simulink model "sampleModel7288_pp_1_1"  (R2018a)
settings: Solver=VariableStepAuto  StartTime=0.0  StopTime=10.0  RelTol=1e-3
undefined symbols (not defined in the file): DiscIntNeverNeededParam, sigbuilder_block
libraries: simulink x497
(part 2 of 10)

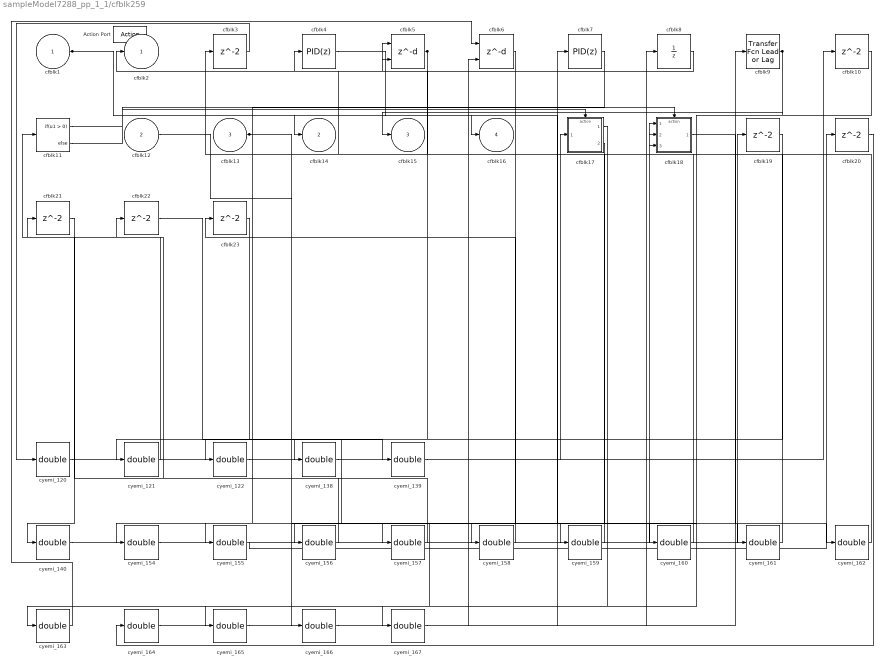
== system sampleModel7288_pp_1_1/cfblk259 ==
  cfblk1 : Inport
  cfblk12 : Inport  Port=2
  cfblk13 : Inport  Port=3
  Action Port : ActionPort  ActionType=else
  cfblk{3,10,19..23} (7 alike) : Delay
  cfblk11 : If  SampleTime=1
  cfblk17 : Subsystem  TreatAsAtomicUnit=on
  cfblk18 : Subsystem  TreatAsAtomicUnit=on
  cfblk4 : simulink/Continuous/PID Controller  Controller=PID  TimeDomain=Discrete-time  SampleTime=-1  IntegratorMethod=Forward Euler  FilterMethod=Forward Euler  Form=Parallel  UseFilter=on  ControllerParametersSource=internal  P=1  I=1  D=0  N=100  InitialConditionSource=internal  InitialConditionForIntegrator=0  InitialConditionForFilter=0  ExternalReset=none  LimitOutput=off  UpperSaturationLimit=inf  LowerSaturationLimit=-inf  LinearizeAsGain=off  AntiWindupMode=none  Kb=1  TrackingMode=off  Kt=1  PParamMin=[]  PParamMax=[]  IParamMin=[]  IParamMax=[]  DParamMin=[]  DParamMax=[]  NParamMin=[]  NParamMax=[]  KbParamMin=[]  KbParamMax=[]  KtParamMin=[]  KtParamMax=[]  POutMin=[]  POutMax=[]  IOutMin=[]  IOutMax=[]  DOutMin=[]  DOutMax=[]  NOutMin=[]  NOutMax=[]  KbOutMin=[]  KbOutMax=[]  KtOutMin=[]  KtOutMax=[]  IntegratorOutMin=[]  IntegratorOutMax=[]  FilterOutMin=[]  FilterOutMax=[]  SumOutMin=[]  SumOutMax=[]  SumI1OutMin=[]  SumI1OutMax=[]  SumI2OutMin=[]  SumI2OutMax=[]  SumI3OutMin=[]  SumI3OutMax=[]  SumDOutMin=[]  SumDOutMax=[]  SaturationOutMin=[]  SaturationOutMax=[]  IntegratorContinuousStateAttributes=''  IntegratorStateMustResolveToSignalObject=off  IntegratorRTWStateStorageClass=Auto  FilterContinuousStateAttributes=''  FilterStateMustResolveToSignalObject=off  FilterRTWStateStorageClass=Auto  DifferentiatorICPrevScaledInput=0  DifferentiatorOutMin=[]  DifferentiatorOutMax=[]  FilterDiffOutCoefMin=[]  FilterDiffOutCoefMax=[]  SumDenOutMin=[]  SumDenOutMax=[]  SumNumOutMin=[]  SumNumOutMax=[]  ReciprocalOutMin=[]  ReciprocalOutMax=[]  DivideOutMin=[]  DivideOutMax=[]  TunerSelectOption=Transfer Function Based (PID Tuner App)
  cfblk5 : Delay  DelayLengthSource=Input port
      settings: InputPortMap=u0,p1
  cfblk6 : Delay  DelayLengthSource=Input port
      settings: InputPortMap=u0,p1
  cfblk7 : simulink/Continuous/PID Controller  Controller=PID  TimeDomain=Discrete-time  SampleTime=-1  IntegratorMethod=Forward Euler  FilterMethod=Forward Euler  Form=Parallel  UseFilter=on  ControllerParametersSource=internal  P=1  I=1  D=0  N=100  InitialConditionSource=internal  InitialConditionForIntegrator=0  InitialConditionForFilter=0  ExternalReset=none  LimitOutput=off  UpperSaturationLimit=inf  LowerSaturationLimit=-inf  LinearizeAsGain=off  AntiWindupMode=none  Kb=1  TrackingMode=off  Kt=1  PParamMin=[]  PParamMax=[]  IParamMin=[]  IParamMax=[]  DParamMin=[]  DParamMax=[]  NParamMin=[]  NParamMax=[]  KbParamMin=[]  KbParamMax=[]  KtParamMin=[]  KtParamMax=[]  POutMin=[]  POutMax=[]  IOutMin=[]  IOutMax=[]  DOutMin=[]  DOutMax=[]  NOutMin=[]  NOutMax=[]  KbOutMin=[]  KbOutMax=[]  KtOutMin=[]  KtOutMax=[]  IntegratorOutMin=[]  IntegratorOutMax=[]  FilterOutMin=[]  FilterOutMax=[]  SumOutMin=[]  SumOutMax=[]  SumI1OutMin=[]  SumI1OutMax=[]  SumI2OutMin=[]  SumI2OutMax=[]  SumI3OutMin=[]  SumI3OutMax=[]  SumDOutMin=[]  SumDOutMax=[]  SaturationOutMin=[]  SaturationOutMax=[]  IntegratorContinuousStateAttributes=''  IntegratorStateMustResolveToSignalObject=off  IntegratorRTWStateStorageClass=Auto  FilterContinuousStateAttributes=''  FilterStateMustResolveToSignalObject=off  FilterRTWStateStorageClass=Auto  DifferentiatorICPrevScaledInput=0  DifferentiatorOutMin=[]  DifferentiatorOutMax=[]  FilterDiffOutCoefMin=[]  FilterDiffOutCoefMax=[]  SumDenOutMin=[]  SumDenOutMax=[]  SumNumOutMin=[]  SumNumOutMax=[]  ReciprocalOutMin=[]  ReciprocalOutMax=[]  DivideOutMin=[]  DivideOutMax=[]  TunerSelectOption=Transfer Function Based (PID Tuner App)
  cfblk8 : UnitDelay  SampleTime=-1
  cfblk9 : simulink/Discrete/Transfer Fcn Lead or Lag  PoleZ=0.95  ZeroZ=0.75  ICPrevOutput=0.0  ICPrevInput=0.0  DoSatur=off
      settings: SourceProductName=Simulink  SourceProductBaseCode=SL
  cyemi_{120..122,138..140,154..167} (20 alike) : DataTypeConversion  OutDataTypeStr=double
  cfblk2 : Outport
  cfblk14 : Outport  Port=2
  cfblk15 : Outport  Port=3
  cfblk16 : Outport  Port=4
  wires:
  cfblk13/1 -> cyemi_159/1, cyemi_160/1
  cfblk8/1 -> cfblk2/1
  cfblk9/1 -> cfblk15/1, cyemi_154/1, cyemi_157/1
  cfblk5/1 -> cyemi_155/1, cyemi_156/1
  cfblk1/1 -> cfblk14/1, cfblk16/1
  cfblk11/1 -> cfblk17/Action
  cfblk11/2 -> cfblk18/Action
  cyemi_120/1 -> cfblk10/1
  cfblk3/1 -> cyemi_120/1
  cyemi_121/1 -> cfblk11/1
  cfblk23/1 -> cyemi_121/1
  cyemi_122/1 -> cfblk17/1(cfblk1)
  cfblk7/1 -> cyemi_122/1
  cyemi_138/1 -> cfblk18/1(cfblk1)
  cfblk19/1 -> cyemi_138/1
  cyemi_139/1 -> cfblk18/2(cfblk12)
  cfblk22/1 -> cyemi_139/1
  cyemi_140/1 -> cfblk18/3(cfblk13)
  cfblk21/1 -> cyemi_140/1
  cyemi_154/1 -> cfblk19/1
  cyemi_155/1 -> cfblk20/1
  cyemi_156/1 -> cfblk21/1
  cyemi_157/1 -> cfblk22/1
  cyemi_158/1 -> cfblk23/1
  cfblk17/2(cfblk11) -> cyemi_158/1
  cyemi_159/1 -> cfblk3/1
  cyemi_160/1 -> cfblk4/1
  cyemi_161/1 -> cfblk5/1
  cfblk4/1 -> cyemi_161/1
  cyemi_162/1 -> cfblk5/2
  cfblk18/1(cfblk2) -> cyemi_162/1
  cyemi_163/1 -> cfblk6/1
  cfblk17/1(cfblk2) -> cyemi_163/1
  cyemi_164/1 -> cfblk6/2
  cfblk20/1 -> cyemi_164/1
  cyemi_165/1 -> cfblk7/1
  cfblk10/1 -> cyemi_165/1
  cyemi_166/1 -> cfblk8/1
  cfblk12/1 -> cyemi_166/1
  cyemi_167/1 -> cfblk9/1
  cfblk6/1 -> cyemi_167/1

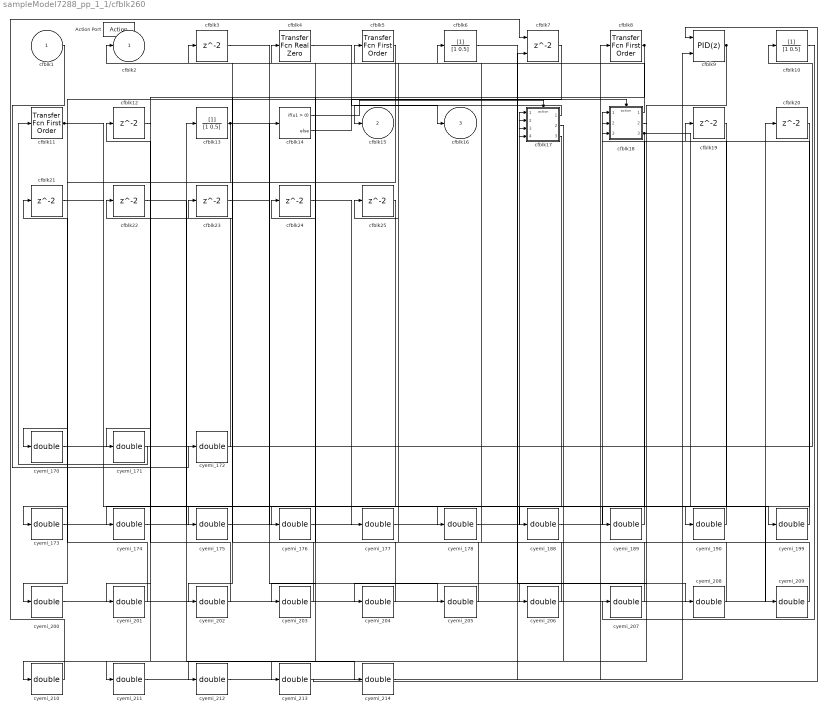
== system sampleModel7288_pp_1_1/cfblk260 ==
  cfblk1 : Inport
  Action Port : ActionPort  ActionType=then
  cfblk10 : DiscreteFilter
  cfblk11 : simulink/Discrete/Transfer Fcn First Order  PoleZ=0.95  ICPrevOutput=0.0  DoSatur=off
      settings: SourceProductName=Simulink
  cfblk{3,12,19..25} (9 alike) : Delay
  cfblk13 : DiscreteFilter
  cfblk14 : If  SampleTime=1
  cfblk17 : Subsystem  TreatAsAtomicUnit=on
  cfblk18 : Subsystem  TreatAsAtomicUnit=on
  cfblk4 : simulink/Discrete/Transfer Fcn Real Zero  ZeroZ=0.75  ICPrevInput=0.0  DoSatur=off
      settings: SourceProductName=Simulink  SourceProductBaseCode=SL
  cfblk5 : simulink/Discrete/Transfer Fcn First Order  PoleZ=0.95  ICPrevOutput=0.0  DoSatur=off
      settings: SourceProductName=Simulink
  cfblk6 : DiscreteFilter
  cfblk7 : Delay  ShowEnablePort=on
      settings: InputPortMap=u0,e6
  cfblk8 : simulink/Discrete/Transfer Fcn First Order  PoleZ=0.95  ICPrevOutput=0.0  DoSatur=off
      settings: SourceProductName=Simulink
  cfblk9 : simulink/Continuous/PID Controller (2DOF)  Controller=PID  TimeDomain=Discrete-time  SampleTime=-1  IntegratorMethod=Forward Euler  FilterMethod=Forward Euler  Form=Parallel  UseFilter=on  ControllerParametersSource=internal  P=1  I=1  D=0  N=100  b=1  c=1  InitialConditionSource=internal  InitialConditionForIntegrator=0  InitialConditionForFilter=0  ExternalReset=none  LimitOutput=off  UpperSaturationLimit=inf  LowerSaturationLimit=-inf  LinearizeAsGain=off  AntiWindupMode=none  Kb=1  TrackingMode=off  Kt=1  PParamMin=[]  PParamMax=[]  IParamMin=[]  IParamMax=[]  DParamMin=[]  DParamMax=[]  NParamMin=[]  NParamMax=[]  bParamMin=[]  bParamMax=[]  cParamMin=[]  cParamMax=[]  KbParamMin=[]  KbParamMax=[]  KtParamMin=[]  KtParamMax=[]  POutMin=[]  POutMax=[]  IOutMin=[]  IOutMax=[]  DOutMin=[]  DOutMax=[]  NOutMin=[]  NOutMax=[]  bOutMin=[]  bOutMax=[]  cOutMin=[]  cOutMax=[]  KbOutMin=[]  KbOutMax=[]  KtOutMin=[]  KtOutMax=[]  IntegratorOutMin=[]  IntegratorOutMax=[]  FilterOutMin=[]  FilterOutMax=[]  SumOutMin=[]  SumOutMax=[]  Sum1OutMin=[]  Sum1OutMax=[]  Sum2OutMin=[]  Sum2OutMax=[]  Sum3OutMin=[]  Sum3OutMax=[]  SumI1OutMin=[]  SumI1OutMax=[]  SumI2OutMin=[]  SumI2OutMax=[]  SumI3OutMin=[]  SumI3OutMax=[]  SumDOutMin=[]  SumDOutMax=[]  SaturationOutMin=[]  SaturationOutMax=[]  IntegratorContinuousStateAttributes=''  IntegratorStateMustResolveToSignalObject=off  IntegratorRTWStateStorageClass=Auto  FilterContinuousStateAttributes=''  FilterStateMustResolveToSignalObject=off  FilterRTWStateStorageClass=Auto  DifferentiatorICPrevScaledInput=0  DifferentiatorOutMin=[]  DifferentiatorOutMax=[]  FilterDiffOutCoefMin=[]  FilterDiffOutCoefMax=[]  SumDenOutMin=[]  SumDenOutMax=[]  SumNumOutMin=[]  SumNumOutMax=[]  ReciprocalOutMin=[]  ReciprocalOutMax=[]  DivideOutMin=[]  DivideOutMax=[]  TunerSelectOption=Transfer Function Based (PID Tuner App)
  cyemi_{170..178,188..190,199..214} (28 alike) : DataTypeConversion  OutDataTypeStr=double
  cfblk2 : Outport
  cfblk15 : Outport  Port=2
  cfblk16 : Outport  Port=3
  wires:
  cfblk9/1 -> cyemi_204/1, cyemi_212/1
  cfblk11/1 -> cyemi_170/1, cyemi_189/1
  cfblk17/1(cfblk2) -> cfblk15/1
  cfblk8/1 -> cyemi_201/1, cyemi_202/1, cyemi_203/1
  cfblk13/1 -> cyemi_199/1, cyemi_200/1
  cfblk18/1(cfblk2) -> cfblk2/1
  cfblk4/1 -> cfblk16/1
  cfblk18/3(cfblk14) -> cyemi_206/1, cyemi_209/1
  cfblk14/1 -> cfblk17/Action
  cfblk14/2 -> cfblk18/Action
  cyemi_170/1 -> cfblk10/1
  cyemi_171/1 -> cfblk11/1
  cfblk12/1 -> cyemi_171/1
  cyemi_172/1 -> cfblk12/1
  cfblk1/1 -> cyemi_172/1
  cyemi_173/1 -> cfblk13/1
  cfblk7/1 -> cyemi_173/1
  cyemi_174/1 -> cfblk14/1
  cfblk25/1 -> cyemi_174/1
  cyemi_175/1 -> cfblk17/1(cfblk1)
  cfblk19/1 -> cyemi_175/1
  cyemi_176/1 -> cfblk17/2(cfblk10)
  cfblk18/2(cfblk13) -> cyemi_176/1
  cyemi_177/1 -> cfblk17/3(cfblk11)
  cfblk24/1 -> cyemi_177/1
  cyemi_178/1 -> cfblk17/4(cfblk12)
  cfblk23/1 -> cyemi_178/1
  cyemi_188/1 -> cfblk18/1(cfblk1)
  cfblk21/1 -> cyemi_188/1
  cyemi_189/1 -> cfblk18/2(cfblk11)
  cyemi_190/1 -> cfblk18/3(cfblk12)
  cfblk20/1 -> cyemi_190/1
  cyemi_199/1 -> cfblk19/1
  cyemi_200/1 -> cfblk20/1
  cyemi_201/1 -> cfblk21/1
  cyemi_202/1 -> cfblk22/1
  cyemi_203/1 -> cfblk23/1
  cyemi_204/1 -> cfblk24/1
  cyemi_205/1 -> cfblk25/1
  cfblk3/1 -> cyemi_205/1
  cyemi_206/1 -> cfblk3/1
  cyemi_207/1 -> cfblk4/1
  cfblk10/1 -> cyemi_207/1
  cyemi_208/1 -> cfblk5/1
  cfblk6/1 -> cyemi_208/1
  cyemi_209/1 -> cfblk6/1
  cyemi_210/1 -> cfblk7/1
  cfblk17/2(cfblk13) -> cyemi_210/1
  cyemi_211/1 -> cfblk7/2
  cfblk5/1 -> cyemi_211/1
  cyemi_212/1 -> cfblk8/1
  cyemi_213/1 -> cfblk9/1
  cfblk17/3(cfblk14) -> cyemi_213/1
  cyemi_214/1 -> cfblk9/2
  cfblk22/1 -> cyemi_214/1

== system sampleModel7288_pp_1_1/cfblk261 ==
  cfblk1 : Inport
  cfblk12 : Inport  Port=2
  Action Port : ActionPort  ActionType=else
  cfblk10 : simulink/Continuous/PID Controller  Controller=PID  TimeDomain=Discrete-time  SampleTime=-1  IntegratorMethod=Forward Euler  FilterMethod=Forward Euler  Form=Parallel  UseFilter=on  ControllerParametersSource=internal  P=1  I=1  D=0  N=100  InitialConditionSource=internal  InitialConditionForIntegrator=0  InitialConditionForFilter=0  ExternalReset=none  LimitOutput=off  UpperSaturationLimit=inf  LowerSaturationLimit=-inf  LinearizeAsGain=off  AntiWindupMode=none  Kb=1  TrackingMode=off  Kt=1  PParamMin=[]  PParamMax=[]  IParamMin=[]  IParamMax=[]  DParamMin=[]  DParamMax=[]  NParamMin=[]  NParamMax=[]  KbParamMin=[]  KbParamMax=[]  KtParamMin=[]  KtParamMax=[]  POutMin=[]  POutMax=[]  IOutMin=[]  IOutMax=[]  DOutMin=[]  DOutMax=[]  NOutMin=[]  NOutMax=[]  KbOutMin=[]  KbOutMax=[]  KtOutMin=[]  KtOutMax=[]  IntegratorOutMin=[]  IntegratorOutMax=[]  FilterOutMin=[]  FilterOutMax=[]  SumOutMin=[]  SumOutMax=[]  SumI1OutMin=[]  SumI1OutMax=[]  SumI2OutMin=[]  SumI2OutMax=[]  SumI3OutMin=[]  SumI3OutMax=[]  SumDOutMin=[]  SumDOutMax=[]  SaturationOutMin=[]  SaturationOutMax=[]  IntegratorContinuousStateAttributes=''  IntegratorStateMustResolveToSignalObject=off  IntegratorRTWStateStorageClass=Auto  FilterContinuousStateAttributes=''  FilterStateMustResolveToSignalObject=off  FilterRTWStateStorageClass=Auto  DifferentiatorICPrevScaledInput=0  DifferentiatorOutMin=[]  DifferentiatorOutMax=[]  FilterDiffOutCoefMin=[]  FilterDiffOutCoefMax=[]  SumDenOutMin=[]  SumDenOutMax=[]  SumNumOutMin=[]  SumNumOutMax=[]  ReciprocalOutMin=[]  ReciprocalOutMax=[]  DivideOutMin=[]  DivideOutMax=[]  TunerSelectOption=Transfer Function Based (PID Tuner App)
  cfblk11 : simulink/Discrete/Transfer Fcn First Order  PoleZ=0.95  ICPrevOutput=0.0  DoSatur=off
      settings: SourceProductName=Simulink
  cfblk16 : Delay
  cfblk17 : Delay
  cfblk3 : simulink/Continuous/PID Controller (2DOF)  Controller=PID  TimeDomain=Discrete-time  SampleTime=-1  IntegratorMethod=Forward Euler  FilterMethod=Forward Euler  Form=Parallel  UseFilter=on  ControllerParametersSource=internal  P=1  I=1  D=0  N=100  b=1  c=1  InitialConditionSource=internal  InitialConditionForIntegrator=0  InitialConditionForFilter=0  ExternalReset=none  LimitOutput=off  UpperSaturationLimit=inf  LowerSaturationLimit=-inf  LinearizeAsGain=off  AntiWindupMode=none  Kb=1  TrackingMode=off  Kt=1  PParamMin=[]  PParamMax=[]  IParamMin=[]  IParamMax=[]  DParamMin=[]  DParamMax=[]  NParamMin=[]  NParamMax=[]  bParamMin=[]  bParamMax=[]  cParamMin=[]  cParamMax=[]  KbParamMin=[]  KbParamMax=[]  KtParamMin=[]  KtParamMax=[]  POutMin=[]  POutMax=[]  IOutMin=[]  IOutMax=[]  DOutMin=[]  DOutMax=[]  NOutMin=[]  NOutMax=[]  bOutMin=[]  bOutMax=[]  cOutMin=[]  cOutMax=[]  KbOutMin=[]  KbOutMax=[]  KtOutMin=[]  KtOutMax=[]  IntegratorOutMin=[]  IntegratorOutMax=[]  FilterOutMin=[]  FilterOutMax=[]  SumOutMin=[]  SumOutMax=[]  Sum1OutMin=[]  Sum1OutMax=[]  Sum2OutMin=[]  Sum2OutMax=[]  Sum3OutMin=[]  Sum3OutMax=[]  SumI1OutMin=[]  SumI1OutMax=[]  SumI2OutMin=[]  SumI2OutMax=[]  SumI3OutMin=[]  SumI3OutMax=[]  SumDOutMin=[]  SumDOutMax=[]  SaturationOutMin=[]  SaturationOutMax=[]  IntegratorContinuousStateAttributes=''  IntegratorStateMustResolveToSignalObject=off  IntegratorRTWStateStorageClass=Auto  FilterContinuousStateAttributes=''  FilterStateMustResolveToSignalObject=off  FilterRTWStateStorageClass=Auto  DifferentiatorICPrevScaledInput=0  DifferentiatorOutMin=[]  DifferentiatorOutMax=[]  FilterDiffOutCoefMin=[]  FilterDiffOutCoefMax=[]  SumDenOutMin=[]  SumDenOutMax=[]  SumNumOutMin=[]  SumNumOutMax=[]  ReciprocalOutMin=[]  ReciprocalOutMax=[]  DivideOutMin=[]  DivideOutMax=[]  TunerSelectOption=Transfer Function Based (PID Tuner App)
  cfblk4 : Delay  ShowEnablePort=on
      settings: InputPortMap=u0,e6
  cfblk5 : Delay
  cfblk6 : DiscreteFir
  cfblk7 : simulink/Continuous/PID Controller (2DOF)  Controller=PID  TimeDomain=Discrete-time  SampleTime=-1  IntegratorMethod=Forward Euler  FilterMethod=Forward Euler  Form=Parallel  UseFilter=on  ControllerParametersSource=internal  P=1  I=1  D=0  N=100  b=1  c=1  InitialConditionSource=internal  InitialConditionForIntegrator=0  InitialConditionForFilter=0  ExternalReset=none  LimitOutput=off  UpperSaturationLimit=inf  LowerSaturationLimit=-inf  LinearizeAsGain=off  AntiWindupMode=none  Kb=1  TrackingMode=off  Kt=1  PParamMin=[]  PParamMax=[]  IParamMin=[]  IParamMax=[]  DParamMin=[]  DParamMax=[]  NParamMin=[]  NParamMax=[]  bParamMin=[]  bParamMax=[]  cParamMin=[]  cParamMax=[]  KbParamMin=[]  KbParamMax=[]  KtParamMin=[]  KtParamMax=[]  POutMin=[]  POutMax=[]  IOutMin=[]  IOutMax=[]  DOutMin=[]  DOutMax=[]  NOutMin=[]  NOutMax=[]  bOutMin=[]  bOutMax=[]  cOutMin=[]  cOutMax=[]  KbOutMin=[]  KbOutMax=[]  KtOutMin=[]  KtOutMax=[]  IntegratorOutMin=[]  IntegratorOutMax=[]  FilterOutMin=[]  FilterOutMax=[]  SumOutMin=[]  SumOutMax=[]  Sum1OutMin=[]  Sum1OutMax=[]  Sum2OutMin=[]  Sum2OutMax=[]  Sum3OutMin=[]  Sum3OutMax=[]  SumI1OutMin=[]  SumI1OutMax=[]  SumI2OutMin=[]  SumI2OutMax=[]  SumI3OutMin=[]  SumI3OutMax=[]  SumDOutMin=[]  SumDOutMax=[]  SaturationOutMin=[]  SaturationOutMax=[]  IntegratorContinuousStateAttributes=''  IntegratorStateMustResolveToSignalObject=off  IntegratorRTWStateStorageClass=Auto  FilterContinuousStateAttributes=''  FilterStateMustResolveToSignalObject=off  FilterRTWStateStorageClass=Auto  DifferentiatorICPrevScaledInput=0  DifferentiatorOutMin=[]  DifferentiatorOutMax=[]  FilterDiffOutCoefMin=[]  FilterDiffOutCoefMax=[]  SumDenOutMin=[]  SumDenOutMax=[]  SumNumOutMin=[]  SumNumOutMax=[]  ReciprocalOutMin=[]  ReciprocalOutMax=[]  DivideOutMin=[]  DivideOutMax=[]  TunerSelectOption=Transfer Function Based (PID Tuner App)
  cfblk8 : simulink/Continuous/PID Controller  Controller=PID  TimeDomain=Discrete-time  SampleTime=-1  IntegratorMethod=Forward Euler  FilterMethod=Forward Euler  Form=Parallel  UseFilter=on  ControllerParametersSource=internal  P=1  I=1  D=0  N=100  InitialConditionSource=internal  InitialConditionForIntegrator=0  InitialConditionForFilter=0  ExternalReset=none  LimitOutput=off  UpperSaturationLimit=inf  LowerSaturationLimit=-inf  LinearizeAsGain=off  AntiWindupMode=none  Kb=1  TrackingMode=off  Kt=1  PParamMin=[]  PParamMax=[]  IParamMin=[]  IParamMax=[]  DParamMin=[]  DParamMax=[]  NParamMin=[]  NParamMax=[]  KbParamMin=[]  KbParamMax=[]  KtParamMin=[]  KtParamMax=[]  POutMin=[]  POutMax=[]  IOutMin=[]  IOutMax=[]  DOutMin=[]  DOutMax=[]  NOutMin=[]  NOutMax=[]  KbOutMin=[]  KbOutMax=[]  KtOutMin=[]  KtOutMax=[]  IntegratorOutMin=[]  IntegratorOutMax=[]  FilterOutMin=[]  FilterOutMax=[]  SumOutMin=[]  SumOutMax=[]  SumI1OutMin=[]  SumI1OutMax=[]  SumI2OutMin=[]  SumI2OutMax=[]  SumI3OutMin=[]  SumI3OutMax=[]  SumDOutMin=[]  SumDOutMax=[]  SaturationOutMin=[]  SaturationOutMax=[]  IntegratorContinuousStateAttributes=''  IntegratorStateMustResolveToSignalObject=off  IntegratorRTWStateStorageClass=Auto  FilterContinuousStateAttributes=''  FilterStateMustResolveToSignalObject=off  FilterRTWStateStorageClass=Auto  DifferentiatorICPrevScaledInput=0  DifferentiatorOutMin=[]  DifferentiatorOutMax=[]  FilterDiffOutCoefMin=[]  FilterDiffOutCoefMax=[]  SumDenOutMin=[]  SumDenOutMax=[]  SumNumOutMin=[]  SumNumOutMax=[]  ReciprocalOutMin=[]  ReciprocalOutMax=[]  DivideOutMin=[]  DivideOutMax=[]  TunerSelectOption=Transfer Function Based (PID Tuner App)
  cfblk9 : simulink/Discrete/Difference  ICPrevInput=0.0  OutMin=[]  OutMax=[]  OutDataTypeStr=double  OutputDataTypeScalingMode=double  OutDataType=fixdt(1, 16)  OutScaling=2^-10  DoSatur=off
  cyemi_{217..230} (14 alike) : DataTypeConversion  OutDataTypeStr=double
  cfblk2 : Outport
  cfblk13 : Outport  Port=2
  cfblk14 : Outport  Port=3
  cfblk15 : Outport  Port=4
  wires:
  cfblk9/1 -> cfblk15/1
  cfblk1/1 -> cyemi_223/1, cyemi_224/1, cyemi_226/1
  cfblk7/1 -> cfblk13/1
  cfblk10/1 -> cyemi_219/1, cyemi_220/1
  cfblk8/1 -> cfblk14/1, cfblk2/1, cyemi_217/1
  cyemi_217/1 -> cfblk10/1
  cyemi_218/1 -> cfblk11/1
  cfblk4/1 -> cyemi_218/1
  cyemi_219/1 -> cfblk16/1
  cyemi_220/1 -> cfblk17/1
  cyemi_221/1 -> cfblk3/1
  cfblk16/1 -> cyemi_221/1
  cyemi_222/1 -> cfblk3/2
  cfblk17/1 -> cyemi_222/1
  cyemi_223/1 -> cfblk4/1
  cyemi_224/1 -> cfblk4/2
  cyemi_225/1 -> cfblk5/1
  cfblk6/1 -> cyemi_225/1
  cyemi_226/1 -> cfblk6/1
  cyemi_227/1 -> cfblk7/1
  cfblk12/1 -> cyemi_227/1
  cyemi_228/1 -> cfblk7/2
  cfblk5/1 -> cyemi_228/1
  cyemi_229/1 -> cfblk8/1
  cfblk3/1 -> cyemi_229/1
  cyemi_230/1 -> cfblk9/1
  cfblk11/1 -> cyemi_230/1

== system sampleModel7288_pp_1_1/cfblk262 ==
  cfblk1 : Inport
  cfblk7 : Inport  Port=2
  Action Port : ActionPort  ActionType=then
  cfblk10 : Delay
  cfblk11 : Delay
  cfblk12 : Delay
  cfblk3 : Delay  ShowEnablePort=on
      settings: InputPortMap=u0,e6
  cfblk4 : DiscreteIntegrator  SampleTime=-1  OutDataTypeStr=double  ICPrevOutput=DiscIntNeverNeededParam  ICPrevScaledInput=DiscIntNeverNeededParam
  cfblk5 : Delay  DelayLengthSource=Input port
      settings: InputPortMap=u0,p1
  cfblk6 : If  SampleTime=1
  cfblk8 : Subsystem  TreatAsAtomicUnit=on
  cfblk9 : Subsystem  TreatAsAtomicUnit=on
  cyemi_{233..243,254..255} (13 alike) : DataTypeConversion  OutDataTypeStr=double
  cfblk2 : Outport
  wires:
  cfblk3/1 -> cfblk2/1, cyemi_242/1
  cfblk6/1 -> cfblk8/Action
  cfblk6/2 -> cfblk9/Action
  cyemi_233/1 -> cfblk10/1
  cfblk5/1 -> cyemi_233/1
  cyemi_234/1 -> cfblk11/1
  cfblk9/2(cfblk15) -> cyemi_234/1
  cyemi_235/1 -> cfblk12/1
  cfblk8/3(cfblk12) -> cyemi_235/1
  cyemi_236/1 -> cfblk3/1
  cfblk1/1 -> cyemi_236/1
  cyemi_237/1 -> cfblk3/2
  cfblk12/1 -> cyemi_237/1
  cyemi_238/1 -> cfblk4/1
  cfblk9/1(cfblk2) -> cyemi_238/1
  cyemi_239/1 -> cfblk5/1
  cfblk7/1 -> cyemi_239/1
  cyemi_240/1 -> cfblk5/2
  cfblk4/1 -> cyemi_240/1
  cyemi_241/1 -> cfblk6/1
  cfblk11/1 -> cyemi_241/1
  cyemi_242/1 -> cfblk8/1(cfblk1)
  cyemi_243/1 -> cfblk8/2(cfblk10)
  cfblk10/1 -> cyemi_243/1
  cyemi_254/1 -> cfblk9/1(cfblk1)
  cfblk8/1(cfblk2) -> cyemi_254/1
  cyemi_255/1 -> cfblk9/2(cfblk14)
  cfblk8/2(cfblk11) -> cyemi_255/1

== system sampleModel7288_pp_1_1/cfblk263 ==
  cfblk1 : Inport
  Action Port : ActionPort  ActionType=else
  cfblk10 : Delay  DelayLengthSource=Input port
      settings: InputPortMap=u0,p1
  cfblk11 : UnitDelay  SampleTime=-1
  cfblk12 : Delay
  cfblk3 : DiscreteIntegrator  SampleTime=-1  OutDataTypeStr=double  ICPrevOutput=DiscIntNeverNeededParam  ICPrevScaledInput=DiscIntNeverNeededParam
  cfblk4 : simulink/Discrete/Transfer Fcn Real Zero  ZeroZ=0.75  ICPrevInput=0.0  DoSatur=off
      settings: SourceProductName=Simulink  SourceProductBaseCode=SL
  cfblk5 : simulink/Discrete/Tapped Delay  vinit=0.0  samptime=-1  NumDelays=1  DelayOrder=Oldest  includeCurrent=off
  cfblk6 : Delay  ShowEnablePort=on
      settings: InputPortMap=u0,e6
  cfblk7 : simulink/Continuous/PID Controller (2DOF)  Controller=PID  TimeDomain=Discrete-time  SampleTime=-1  IntegratorMethod=Forward Euler  FilterMethod=Forward Euler  Form=Parallel  UseFilter=on  ControllerParametersSource=internal  P=1  I=1  D=0  N=100  b=1  c=1  InitialConditionSource=internal  InitialConditionForIntegrator=0  InitialConditionForFilter=0  ExternalReset=none  LimitOutput=off  UpperSaturationLimit=inf  LowerSaturationLimit=-inf  LinearizeAsGain=off  AntiWindupMode=none  Kb=1  TrackingMode=off  Kt=1  PParamMin=[]  PParamMax=[]  IParamMin=[]  IParamMax=[]  DParamMin=[]  DParamMax=[]  NParamMin=[]  NParamMax=[]  bParamMin=[]  bParamMax=[]  cParamMin=[]  cParamMax=[]  KbParamMin=[]  KbParamMax=[]  KtParamMin=[]  KtParamMax=[]  POutMin=[]  POutMax=[]  IOutMin=[]  IOutMax=[]  DOutMin=[]  DOutMax=[]  NOutMin=[]  NOutMax=[]  bOutMin=[]  bOutMax=[]  cOutMin=[]  cOutMax=[]  KbOutMin=[]  KbOutMax=[]  KtOutMin=[]  KtOutMax=[]  IntegratorOutMin=[]  IntegratorOutMax=[]  FilterOutMin=[]  FilterOutMax=[]  SumOutMin=[]  SumOutMax=[]  Sum1OutMin=[]  Sum1OutMax=[]  Sum2OutMin=[]  Sum2OutMax=[]  Sum3OutMin=[]  Sum3OutMax=[]  SumI1OutMin=[]  SumI1OutMax=[]  SumI2OutMin=[]  SumI2OutMax=[]  SumI3OutMin=[]  SumI3OutMax=[]  SumDOutMin=[]  SumDOutMax=[]  SaturationOutMin=[]  SaturationOutMax=[]  IntegratorContinuousStateAttributes=''  IntegratorStateMustResolveToSignalObject=off  IntegratorRTWStateStorageClass=Auto  FilterContinuousStateAttributes=''  FilterStateMustResolveToSignalObject=off  FilterRTWStateStorageClass=Auto  DifferentiatorICPrevScaledInput=0  DifferentiatorOutMin=[]  DifferentiatorOutMax=[]  FilterDiffOutCoefMin=[]  FilterDiffOutCoefMax=[]  SumDenOutMin=[]  SumDenOutMax=[]  SumNumOutMin=[]  SumNumOutMax=[]  ReciprocalOutMin=[]  ReciprocalOutMax=[]  DivideOutMin=[]  DivideOutMax=[]  TunerSelectOption=Transfer Function Based (PID Tuner App)
  cfblk8 : simulink/Discrete/Difference  ICPrevInput=0.0  OutMin=[]  OutMax=[]  OutDataTypeStr=double  OutputDataTypeScalingMode=double  OutDataType=fixdt(1, 16)  OutScaling=2^-10  DoSatur=off
  cfblk9 : Delay
  cyemi_{271..283} (13 alike) : DataTypeConversion  OutDataTypeStr=double
  cfblk2 : Outport
  wires:
  cfblk1/1 -> cyemi_280/1, cyemi_282/1
  cfblk11/1 -> cyemi_277/1, cyemi_281/1
  cfblk3/1 -> cfblk2/1
  cyemi_271/1 -> cfblk10/1
  cfblk6/1 -> cyemi_271/1, cyemi_272/1
  cyemi_272/1 -> cfblk10/2
  cyemi_273/1 -> cfblk11/1
  cfblk4/1 -> cyemi_273/1
  cyemi_274/1 -> cfblk12/1
  cfblk10/1 -> cyemi_274/1
  cyemi_275/1 -> cfblk3/1
  cfblk5/1 -> cyemi_275/1
  cyemi_276/1 -> cfblk4/1
  cfblk9/1 -> cyemi_276/1
  cyemi_277/1 -> cfblk5/1
  cyemi_278/1 -> cfblk6/1
  cfblk12/1 -> cyemi_278/1
  cyemi_279/1 -> cfblk6/2
  cfblk7/1 -> cyemi_279/1
  cyemi_280/1 -> cfblk7/1
  cyemi_281/1 -> cfblk7/2
  cyemi_282/1 -> cfblk8/1
  cyemi_283/1 -> cfblk9/1
  cfblk8/1 -> cyemi_283/1

== system sampleModel7288_pp_1_1/cfblk264 ==
  cfblk1 : Inport
  Action Port : ActionPort  ActionType=then
  cfblk10 : simulink/Discrete/Transfer Fcn Lead or Lag  PoleZ=0.95  ZeroZ=0.75  ICPrevOutput=0.0  ICPrevInput=0.0  DoSatur=off
      settings: SourceProductName=Simulink  SourceProductBaseCode=SL
  cfblk11 : simulink/Discrete/Transfer Fcn Real Zero  ZeroZ=0.75  ICPrevInput=0.0  DoSatur=off
      settings: SourceProductName=Simulink  SourceProductBaseCode=SL
  cfblk12 : DiscreteIntegrator  SampleTime=-1  OutDataTypeStr=double  ICPrevOutput=DiscIntNeverNeededParam  ICPrevScaledInput=DiscIntNeverNeededParam
  cfblk13 : DiscreteFir
  cfblk16 : Delay
  cfblk17 : Delay
  cfblk3 : simulink/Discrete/Difference  ICPrevInput=0.0  OutMin=[]  OutMax=[]  OutDataTypeStr=double  OutputDataTypeScalingMode=double  OutDataType=fixdt(1, 16)  OutScaling=2^-10  DoSatur=off
  cfblk4 : DiscreteZeroPole  Poles=[0 0.5]  Gain=1  SampleTime=-1
  cfblk5 : Delay  DelayLengthSource=Input port
      settings: InputPortMap=u0,p1
  cfblk6 : simulink/Continuous/PID Controller (2DOF)  Controller=PID  TimeDomain=Discrete-time  SampleTime=-1  IntegratorMethod=Forward Euler  FilterMethod=Forward Euler  Form=Parallel  UseFilter=on  ControllerParametersSource=internal  P=1  I=1  D=0  N=100  b=1  c=1  InitialConditionSource=internal  InitialConditionForIntegrator=0  InitialConditionForFilter=0  ExternalReset=none  LimitOutput=off  UpperSaturationLimit=inf  LowerSaturationLimit=-inf  LinearizeAsGain=off  AntiWindupMode=none  Kb=1  TrackingMode=off  Kt=1  PParamMin=[]  PParamMax=[]  IParamMin=[]  IParamMax=[]  DParamMin=[]  DParamMax=[]  NParamMin=[]  NParamMax=[]  bParamMin=[]  bParamMax=[]  cParamMin=[]  cParamMax=[]  KbParamMin=[]  KbParamMax=[]  KtParamMin=[]  KtParamMax=[]  POutMin=[]  POutMax=[]  IOutMin=[]  IOutMax=[]  DOutMin=[]  DOutMax=[]  NOutMin=[]  NOutMax=[]  bOutMin=[]  bOutMax=[]  cOutMin=[]  cOutMax=[]  KbOutMin=[]  KbOutMax=[]  KtOutMin=[]  KtOutMax=[]  IntegratorOutMin=[]  IntegratorOutMax=[]  FilterOutMin=[]  FilterOutMax=[]  SumOutMin=[]  SumOutMax=[]  Sum1OutMin=[]  Sum1OutMax=[]  Sum2OutMin=[]  Sum2OutMax=[]  Sum3OutMin=[]  Sum3OutMax=[]  SumI1OutMin=[]  SumI1OutMax=[]  SumI2OutMin=[]  SumI2OutMax=[]  SumI3OutMin=[]  SumI3OutMax=[]  SumDOutMin=[]  SumDOutMax=[]  SaturationOutMin=[]  SaturationOutMax=[]  IntegratorContinuousStateAttributes=''  IntegratorStateMustResolveToSignalObject=off  IntegratorRTWStateStorageClass=Auto  FilterContinuousStateAttributes=''  FilterStateMustResolveToSignalObject=off  FilterRTWStateStorageClass=Auto  DifferentiatorICPrevScaledInput=0  DifferentiatorOutMin=[]  DifferentiatorOutMax=[]  FilterDiffOutCoefMin=[]  FilterDiffOutCoefMax=[]  SumDenOutMin=[]  SumDenOutMax=[]  SumNumOutMin=[]  SumNumOutMax=[]  ReciprocalOutMin=[]  ReciprocalOutMax=[]  DivideOutMin=[]  DivideOutMax=[]  TunerSelectOption=Transfer Function Based (PID Tuner App)
  cfblk7 : DiscreteFilter
  cfblk8 : UnitDelay  SampleTime=-1
  cfblk9 : DiscreteIntegrator  SampleTime=-1  OutDataTypeStr=double  ICPrevOutput=DiscIntNeverNeededParam  ICPrevScaledInput=DiscIntNeverNeededParam
  cyemi_{285..299} (15 alike) : DataTypeConversion  OutDataTypeStr=double
  cfblk2 : Outport
  cfblk14 : Outport  Port=2
  cfblk15 : Outport  Port=3
  wires:
  cfblk8/1 -> cfblk14/1, cyemi_289/1, cyemi_292/1
  cfblk1/1 -> cyemi_288/1, cyemi_294/1
  cfblk9/1 -> cyemi_285/1, cyemi_290/1
  cfblk12/1 -> cfblk15/1
  cfblk5/1 -> cfblk2/1
  cyemi_285/1 -> cfblk10/1
  cyemi_286/1 -> cfblk11/1
  cfblk10/1 -> cyemi_286/1
  cyemi_287/1 -> cfblk12/1
  cfblk11/1 -> cyemi_287/1
  cyemi_288/1 -> cfblk13/1
  cyemi_289/1 -> cfblk16/1
  cyemi_290/1 -> cfblk17/1
  cyemi_291/1 -> cfblk3/1
  cfblk16/1 -> cyemi_291/1
  cyemi_292/1 -> cfblk4/1
  cyemi_293/1 -> cfblk5/1
  cfblk13/1 -> cyemi_293/1
  cyemi_294/1 -> cfblk5/2
  cyemi_295/1 -> cfblk6/1
  cfblk7/1 -> cyemi_295/1
  cyemi_296/1 -> cfblk6/2
  cfblk17/1 -> cyemi_296/1
  cyemi_297/1 -> cfblk7/1
  cfblk3/1 -> cyemi_297/1
  cyemi_298/1 -> cfblk8/1
  cfblk6/1 -> cyemi_298/1
  cyemi_299/1 -> cfblk9/1
  cfblk4/1 -> cyemi_299/1

== system sampleModel7288_pp_1_1/cfblk265 ==
  cfblk1 : Inport
  cfblk8 : Inport  Port=2
  Action Port : ActionPort  ActionType=else
  cfblk12 : Subsystem  TreatAsAtomicUnit=on
  cfblk13 : Subsystem  TreatAsAtomicUnit=on
  cfblk14 : Delay
  cfblk15 : Delay
  cfblk3 : DiscreteTransferFcn
  cfblk4 : DiscreteZeroPole  Poles=[0 0.5]  Gain=1  SampleTime=-1
  cfblk5 : Delay  ShowEnablePort=on
      settings: InputPortMap=u0,e6
  cfblk6 : simulink/Discrete/Transfer Fcn First Order  PoleZ=0.95  ICPrevOutput=0.0  DoSatur=off
      settings: SourceProductName=Simulink
  cfblk7 : If  SampleTime=1
  cyemi_{302..305,313..314,322..329} (14 alike) : DataTypeConversion  OutDataTypeStr=double
  cfblk2 : Outport
  cfblk9 : Outport  Port=2
  cfblk10 : Outport  Port=3
  cfblk11 : Outport  Port=4
  wires:
  cfblk1/1 -> cfblk10/1, cyemi_303/1, cyemi_325/1
  cfblk6/1 -> cfblk2/1, cyemi_323/1
  cfblk13/1(cfblk2) -> cyemi_304/1, cyemi_305/1, cyemi_324/1
  cfblk12/1(cfblk2) -> cfblk11/1
  cfblk12/3(cfblk14) -> cfblk9/1, cyemi_327/1
  cfblk7/1 -> cfblk12/Action
  cfblk7/2 -> cfblk13/Action
  cyemi_302/1 -> cfblk12/1(cfblk1)
  cfblk14/1 -> cyemi_302/1
  cyemi_303/1 -> cfblk12/2(cfblk10)
  cyemi_304/1 -> cfblk12/3(cfblk11)
  cyemi_305/1 -> cfblk12/4(cfblk12)
  cyemi_313/1 -> cfblk13/1(cfblk1)
  cfblk8/1 -> cyemi_313/1
  cyemi_314/1 -> cfblk13/2(cfblk9)
  cfblk4/1 -> cyemi_314/1
  cyemi_322/1 -> cfblk14/1
  cfblk3/1 -> cyemi_322/1
  cyemi_323/1 -> cfblk15/1
  cyemi_324/1 -> cfblk3/1
  cyemi_325/1 -> cfblk4/1
  cyemi_326/1 -> cfblk5/1
  cfblk12/2(cfblk13) -> cyemi_326/1
  cyemi_327/1 -> cfblk5/2
  cyemi_328/1 -> cfblk6/1
  cfblk5/1 -> cyemi_328/1
  cyemi_329/1 -> cfblk7/1
  cfblk15/1 -> cyemi_329/1

== system sampleModel7288_pp_1_1/cfblk266 ==
  cfblk1 : Inport
  Action Port : ActionPort  ActionType=then
  cfblk3 : DiscreteTransferFcn
  cfblk4 : DiscreteZeroPole  Poles=[0 0.5]  Gain=1  SampleTime=-1
  cfblk5 : DiscreteZeroPole  Poles=[0 0.5]  Gain=1  SampleTime=-1
  cyemi_331 : DataTypeConversion  OutDataTypeStr=double
  cyemi_332 : DataTypeConversion  OutDataTypeStr=double
  cyemi_333 : DataTypeConversion  OutDataTypeStr=double
  cfblk2 : Outport
  cfblk6 : Outport  Port=2
  cfblk7 : Outport  Port=3
  wires:
  cfblk3/1 -> cfblk7/1
  cfblk4/1 -> cfblk2/1, cyemi_333/1
  cfblk1/1 -> cfblk6/1, cyemi_332/1
  cyemi_331/1 -> cfblk3/1
  cfblk5/1 -> cyemi_331/1
  cyemi_332/1 -> cfblk4/1
  cyemi_333/1 -> cfblk5/1

== system sampleModel7288_pp_1_1/cfblk267 ==
  cfblk1 : Inport
  cfblk15 : Inport  Port=2
  cfblk16 : Inport  Port=3
  Action Port : ActionPort  ActionType=else
  cfblk10 : DiscreteFir
  cfblk11 : simulink/Discrete/Transfer Fcn First Order  PoleZ=0.95  ICPrevOutput=0.0  DoSatur=off
      settings: SourceProductName=Simulink
  cfblk12 : Delay  ShowEnablePort=on
      settings: InputPortMap=u0,e6
  cfblk13 : DiscreteTransferFcn
  cfblk14 : simulink/Continuous/PID Controller (2DOF)  Controller=PID  TimeDomain=Discrete-time  SampleTime=-1  IntegratorMethod=Forward Euler  FilterMethod=Forward Euler  Form=Parallel  UseFilter=on  ControllerParametersSource=internal  P=1  I=1  D=0  N=100  b=1  c=1  InitialConditionSource=internal  InitialConditionForIntegrator=0  InitialConditionForFilter=0  ExternalReset=none  LimitOutput=off  UpperSaturationLimit=inf  LowerSaturationLimit=-inf  LinearizeAsGain=off  AntiWindupMode=none  Kb=1  TrackingMode=off  Kt=1  PParamMin=[]  PParamMax=[]  IParamMin=[]  IParamMax=[]  DParamMin=[]  DParamMax=[]  NParamMin=[]  NParamMax=[]  bParamMin=[]  bParamMax=[]  cParamMin=[]  cParamMax=[]  KbParamMin=[]  KbParamMax=[]  KtParamMin=[]  KtParamMax=[]  POutMin=[]  POutMax=[]  IOutMin=[]  IOutMax=[]  DOutMin=[]  DOutMax=[]  NOutMin=[]  NOutMax=[]  bOutMin=[]  bOutMax=[]  cOutMin=[]  cOutMax=[]  KbOutMin=[]  KbOutMax=[]  KtOutMin=[]  KtOutMax=[]  IntegratorOutMin=[]  IntegratorOutMax=[]  FilterOutMin=[]  FilterOutMax=[]  SumOutMin=[]  SumOutMax=[]  Sum1OutMin=[]  Sum1OutMax=[]  Sum2OutMin=[]  Sum2OutMax=[]  Sum3OutMin=[]  Sum3OutMax=[]  SumI1OutMin=[]  SumI1OutMax=[]  SumI2OutMin=[]  SumI2OutMax=[]  SumI3OutMin=[]  SumI3OutMax=[]  SumDOutMin=[]  SumDOutMax=[]  SaturationOutMin=[]  SaturationOutMax=[]  IntegratorContinuousStateAttributes=''  IntegratorStateMustResolveToSignalObject=off  IntegratorRTWStateStorageClass=Auto  FilterContinuousStateAttributes=''  FilterStateMustResolveToSignalObject=off  FilterRTWStateStorageClass=Auto  DifferentiatorICPrevScaledInput=0  DifferentiatorOutMin=[]  DifferentiatorOutMax=[]  FilterDiffOutCoefMin=[]  FilterDiffOutCoefMax=[]  SumDenOutMin=[]  SumDenOutMax=[]  SumNumOutMin=[]  SumNumOutMax=[]  ReciprocalOutMin=[]  ReciprocalOutMax=[]  DivideOutMin=[]  DivideOutMax=[]  TunerSelectOption=Transfer Function Based (PID Tuner App)
  cfblk18 : Delay
  cfblk3 : simulink/Discrete/Transfer Fcn Real Zero  ZeroZ=0.75  ICPrevInput=0.0  DoSatur=off
      settings: SourceProductName=Simulink  SourceProductBaseCode=SL
  cfblk4 : simulink/Discrete/Transfer Fcn Real Zero  ZeroZ=0.75  ICPrevInput=0.0  DoSatur=off
      settings: SourceProductName=Simulink  SourceProductBaseCode=SL
  cfblk5 : DiscreteTransferFcn
  cfblk6 : DiscreteFir
  cfblk7 : DiscreteStateSpace  SampleTime=-1
  cfblk8 : UnitDelay  SampleTime=-1
  cfblk9 : simulink/Discrete/Tapped Delay  vinit=0.0  samptime=-1  NumDelays=1  DelayOrder=Oldest  includeCurrent=off
  cyemi_{337..351} (15 alike) : DataTypeConversion  OutDataTypeStr=double
  cfblk2 : Outport
  cfblk17 : Outport  Port=2
  wires:
  cfblk13/1 -> cfblk2/1
  cfblk9/1 -> cfblk17/1
  cfblk7/1 -> cyemi_341/1, cyemi_345/1
  cyemi_337/1 -> cfblk10/1
  cfblk15/1 -> cyemi_337/1
  cyemi_338/1 -> cfblk11/1
  cfblk14/1 -> cyemi_338/1
  cyemi_339/1 -> cfblk12/1
  cfblk1/1 -> cyemi_339/1
  cyemi_340/1 -> cfblk12/2
  cfblk18/1 -> cyemi_340/1
  cyemi_341/1 -> cfblk13/1
  cyemi_342/1 -> cfblk14/1
  cfblk16/1 -> cyemi_342/1
  cyemi_343/1 -> cfblk14/2
  cfblk8/1 -> cyemi_343/1
  cyemi_344/1 -> cfblk18/1
  cfblk3/1 -> cyemi_344/1
  cyemi_345/1 -> cfblk3/1
  cyemi_346/1 -> cfblk4/1
  cfblk10/1 -> cyemi_346/1
  cyemi_347/1 -> cfblk5/1
  cfblk11/1 -> cyemi_347/1
  cyemi_348/1 -> cfblk6/1
  cfblk12/1 -> cyemi_348/1
  cyemi_349/1 -> cfblk7/1
  cfblk5/1 -> cyemi_349/1
  cyemi_350/1 -> cfblk8/1
  cfblk6/1 -> cyemi_350/1
  cyemi_351/1 -> cfblk9/1
  cfblk4/1 -> cyemi_351/1

== system sampleModel7288_pp_1_1/cfblk268 ==
  cfblk1 : Inport
  Action Port : ActionPort  ActionType=then
  cfblk11 : Subsystem  TreatAsAtomicUnit=on
  cfblk12 : Subsystem  TreatAsAtomicUnit=on
  cfblk13 : Subsystem  TreatAsAtomicUnit=on
  cfblk14 : Subsystem  TreatAsAtomicUnit=on
  cfblk{15..18} (4 alike) : Delay
  cfblk3 : DiscreteZeroPole  Poles=[0 0.5]  Gain=1  SampleTime=-1
  cfblk4 : simulink/Discrete/Transfer Fcn First Order  PoleZ=0.95  ICPrevOutput=0.0  DoSatur=off
      settings: SourceProductName=Simulink
  cfblk5 : DiscreteFilter
  cfblk6 : simulink/Discrete/Transfer Fcn Real Zero  ZeroZ=0.75  ICPrevInput=0.0  DoSatur=off
      settings: SourceProductName=Simulink  SourceProductBaseCode=SL
  cfblk7 : DiscreteTransferFcn
  cfblk8 : If  SampleTime=1
  cfblk9 : If  SampleTime=1
  cyemi_{353..354,364..366,379..380,389,402..412} (19 alike) : DataTypeConversion  OutDataTypeStr=double
  cfblk2 : Outport
  cfblk10 : Outport  Port=2
  wires:
  cfblk6/1 -> cfblk10/1
  cfblk14/3(cfblk15) -> cfblk2/1
  cfblk8/1 -> cfblk11/Action
  cfblk8/2 -> cfblk12/Action
  cfblk9/1 -> cfblk13/Action
  cfblk9/2 -> cfblk14/Action
  cyemi_353/1 -> cfblk11/1(cfblk1)
  cfblk12/2(cfblk15) -> cyemi_353/1
  cyemi_354/1 -> cfblk11/2(cfblk11)
  cfblk12/3(cfblk16) -> cyemi_354/1
  cyemi_364/1 -> cfblk12/1(cfblk1)
  cfblk13/3(cfblk11) -> cyemi_364/1
  cyemi_365/1 -> cfblk12/2(cfblk13)
  cfblk16/1 -> cyemi_365/1
  cyemi_366/1 -> cfblk12/3(cfblk14)
  cfblk4/1 -> cyemi_366/1
  cyemi_379/1 -> cfblk13/1(cfblk1)
  cfblk17/1 -> cyemi_379/1
  cyemi_380/1 -> cfblk13/2(cfblk9)
  cfblk5/1 -> cyemi_380/1
  cyemi_389/1 -> cfblk14/1(cfblk1)
  cfblk18/1 -> cyemi_389/1
  cyemi_402/1 -> cfblk15/1
  cfblk12/1(cfblk2) -> cyemi_402/1
  cyemi_403/1 -> cfblk16/1
  cfblk14/1(cfblk2) -> cyemi_403/1
  cyemi_404/1 -> cfblk17/1
  cfblk14/2(cfblk14) -> cyemi_404/1
  cyemi_405/1 -> cfblk18/1
  cfblk11/1(cfblk2) -> cyemi_405/1
  cyemi_406/1 -> cfblk3/1
  cfblk11/2(cfblk12) -> cyemi_406/1
  cyemi_407/1 -> cfblk4/1
  cfblk13/1(cfblk2) -> cyemi_407/1
  cyemi_408/1 -> cfblk5/1
  cfblk1/1 -> cyemi_408/1
  cyemi_409/1 -> cfblk6/1
  cfblk3/1 -> cyemi_409/1
  cyemi_410/1 -> cfblk7/1
  cfblk13/2(cfblk10) -> cyemi_410/1
  cyemi_411/1 -> cfblk8/1
  cfblk7/1 -> cyemi_411/1
  cyemi_412/1 -> cfblk9/1
  cfblk15/1 -> cyemi_412/1

== system sampleModel7288_pp_1_1/cfblk269 ==
  cfblk1 : Inport
  cfblk14 : Inport  Port=2
  Action Port : ActionPort  ActionType=else
  cfblk10 : simulink/Discrete/Difference  ICPrevInput=0.0  OutMin=[]  OutMax=[]  OutDataTypeStr=double  OutputDataTypeScalingMode=double  OutDataType=fixdt(1, 16)  OutScaling=2^-10  DoSatur=off
  cfblk11 : DiscreteFilter
  cfblk12 : DiscreteZeroPole  Poles=[0 0.5]  Gain=1  SampleTime=-1
  cfblk13 : simulink/Discrete/Transfer Fcn Lead or Lag  PoleZ=0.95  ZeroZ=0.75  ICPrevOutput=0.0  ICPrevInput=0.0  DoSatur=off
      settings: SourceProductName=Simulink  SourceProductBaseCode=SL
  cfblk18 : Delay
  cfblk19 : Delay
  cfblk3 : Delay  DelayLengthSource=Input port
      settings: InputPortMap=u0,p1
  cfblk4 : DiscreteTransferFcn
  cfblk5 : DiscreteStateSpace  SampleTime=-1
  cfblk6 : simulink/Discrete/Transfer Fcn Real Zero  ZeroZ=0.75  ICPrevInput=0.0  DoSatur=off
      settings: SourceProductName=Simulink  SourceProductBaseCode=SL
  cfblk7 : DiscreteFilter
  cfblk8 : Delay  ShowEnablePort=on
      settings: InputPortMap=u0,e6
  cfblk9 : DiscreteIntegrator  SampleTime=-1  OutDataTypeStr=double  ICPrevOutput=DiscIntNeverNeededParam  ICPrevScaledInput=DiscIntNeverNeededParam
  cyemi_{415..429} (15 alike) : DataTypeConversion  OutDataTypeStr=double
  cfblk2 : Outport
  cfblk15 : Outport  Port=2
  cfblk16 : Outport  Port=3
  cfblk17 : Outport  Port=4
  wires:
  cfblk6/1 -> cfblk2/1, cyemi_424/1
  cfblk9/1 -> cfblk15/1, cfblk17/1
  cfblk7/1 -> cyemi_425/1, cyemi_428/1
  cfblk11/1 -> cyemi_417/1, cyemi_429/1
  cfblk14/1 -> cfblk16/1
  cyemi_415/1 -> cfblk10/1
  cfblk1/1 -> cyemi_415/1
  cyemi_416/1 -> cfblk11/1
  cfblk8/1 -> cyemi_416/1
  cyemi_417/1 -> cfblk12/1
  cyemi_418/1 -> cfblk13/1
  cfblk4/1 -> cyemi_418/1
  cyemi_419/1 -> cfblk18/1
  cfblk12/1 -> cyemi_419/1
  cyemi_420/1 -> cfblk19/1
  cfblk13/1 -> cyemi_420/1
  cyemi_421/1 -> cfblk3/1
  cfblk18/1 -> cyemi_421/1
  cyemi_422/1 -> cfblk3/2
  cfblk5/1 -> cyemi_422/1
  cyemi_423/1 -> cfblk4/1
  cfblk19/1 -> cyemi_423/1
  cyemi_424/1 -> cfblk5/1
  cyemi_425/1 -> cfblk6/1
  cyemi_426/1 -> cfblk7/1
  cfblk10/1 -> cyemi_426/1
  cyemi_427/1 -> cfblk8/1
  cfblk3/1 -> cyemi_427/1
  cyemi_428/1 -> cfblk8/2
  cyemi_429/1 -> cfblk9/1

== system sampleModel7288_pp_1_1/cfblk270 ==
  cfblk1 : Inport
  cfblk10 : Inport  Port=2
  cfblk11 : Inport  Port=3
  cfblk12 : Inport  Port=4
  cfblk13 : Inport  Port=5
  Action Port : ActionPort  ActionType=then
  cfblk3 : UnitDelay  SampleTime=-1
  cfblk4 : simulink/Continuous/PID Controller  Controller=PID  TimeDomain=Discrete-time  SampleTime=-1  IntegratorMethod=Forward Euler  FilterMethod=Forward Euler  Form=Parallel  UseFilter=on  ControllerParametersSource=internal  P=1  I=1  D=0  N=100  InitialConditionSource=internal  InitialConditionForIntegrator=0  InitialConditionForFilter=0  ExternalReset=none  LimitOutput=off  UpperSaturationLimit=inf  LowerSaturationLimit=-inf  LinearizeAsGain=off  AntiWindupMode=none  Kb=1  TrackingMode=off  Kt=1  PParamMin=[]  PParamMax=[]  IParamMin=[]  IParamMax=[]  DParamMin=[]  DParamMax=[]  NParamMin=[]  NParamMax=[]  KbParamMin=[]  KbParamMax=[]  KtParamMin=[]  KtParamMax=[]  POutMin=[]  POutMax=[]  IOutMin=[]  IOutMax=[]  DOutMin=[]  DOutMax=[]  NOutMin=[]  NOutMax=[]  KbOutMin=[]  KbOutMax=[]  KtOutMin=[]  KtOutMax=[]  IntegratorOutMin=[]  IntegratorOutMax=[]  FilterOutMin=[]  FilterOutMax=[]  SumOutMin=[]  SumOutMax=[]  SumI1OutMin=[]  SumI1OutMax=[]  SumI2OutMin=[]  SumI2OutMax=[]  SumI3OutMin=[]  SumI3OutMax=[]  SumDOutMin=[]  SumDOutMax=[]  SaturationOutMin=[]  SaturationOutMax=[]  IntegratorContinuousStateAttributes=''  IntegratorStateMustResolveToSignalObject=off  IntegratorRTWStateStorageClass=Auto  FilterContinuousStateAttributes=''  FilterStateMustResolveToSignalObject=off  FilterRTWStateStorageClass=Auto  DifferentiatorICPrevScaledInput=0  DifferentiatorOutMin=[]  DifferentiatorOutMax=[]  FilterDiffOutCoefMin=[]  FilterDiffOutCoefMax=[]  SumDenOutMin=[]  SumDenOutMax=[]  SumNumOutMin=[]  SumNumOutMax=[]  ReciprocalOutMin=[]  ReciprocalOutMax=[]  DivideOutMin=[]  DivideOutMax=[]  TunerSelectOption=Transfer Function Based (PID Tuner App)
  cfblk5 : simulink/Discrete/Tapped Delay  vinit=0.0  samptime=-1  NumDelays=1  DelayOrder=Oldest  includeCurrent=off
  cfblk6 : DiscreteIntegrator  SampleTime=-1  OutDataTypeStr=double  ICPrevOutput=DiscIntNeverNeededParam  ICPrevScaledInput=DiscIntNeverNeededParam
  cfblk7 : simulink/Discrete/Tapped Delay  vinit=0.0  samptime=-1  NumDelays=1  DelayOrder=Oldest  includeCurrent=off
  cfblk8 : Delay  ShowEnablePort=on
      settings: InputPortMap=u0,e6
  cfblk9 : DiscreteFir
  cyemi_{436..443} (8 alike) : DataTypeConversion  OutDataTypeStr=double
  cfblk2 : Outport
  cfblk14 : Outport  Port=2
  cfblk15 : Outport  Port=3
  wires:
  cfblk5/1 -> cfblk2/1
  cfblk3/1 -> cfblk15/1
  cfblk8/1 -> cfblk14/1
  cyemi_436/1 -> cfblk3/1
  cfblk11/1 -> cyemi_436/1
  cyemi_437/1 -> cfblk4/1
  cfblk7/1 -> cyemi_437/1
  cyemi_438/1 -> cfblk5/1
  cfblk6/1 -> cyemi_438/1
  cyemi_439/1 -> cfblk6/1
  cfblk10/1 -> cyemi_439/1
  cyemi_440/1 -> cfblk7/1
  cfblk13/1 -> cyemi_440/1
  cyemi_441/1 -> cfblk8/1
  cfblk4/1 -> cyemi_441/1
  cyemi_442/1 -> cfblk8/2
  cfblk9/1 -> cyemi_442/1
  cyemi_443/1 -> cfblk9/1
  cfblk1/1 -> cyemi_443/1

== system sampleModel7288_pp_1_1/cfblk271 ==
  cfblk1 : Inport
  cfblk11 : Inport  Port=2
  cfblk12 : Inport  Port=3
  cfblk13 : Inport  Port=4
  Action Port : ActionPort  ActionType=else
  cfblk10 : DiscreteZeroPole  Poles=[0 0.5]  Gain=1  SampleTime=-1
  cfblk3 : UnitDelay  SampleTime=-1
  cfblk4 : DiscreteFir
  cfblk5 : DiscreteStateSpace  SampleTime=-1
  cfblk6 : simulink/Discrete/Transfer Fcn First Order  PoleZ=0.95  ICPrevOutput=0.0  DoSatur=off
      settings: SourceProductName=Simulink
  cfblk7 : UnitDelay  SampleTime=-1
  cfblk8 : DiscreteFir
  cfblk9 : simulink/Continuous/PID Controller (2DOF)  Controller=PID  TimeDomain=Discrete-time  SampleTime=-1  IntegratorMethod=Forward Euler  FilterMethod=Forward Euler  Form=Parallel  UseFilter=on  ControllerParametersSource=internal  P=1  I=1  D=0  N=100  b=1  c=1  InitialConditionSource=internal  InitialConditionForIntegrator=0  InitialConditionForFilter=0  ExternalReset=none  LimitOutput=off  UpperSaturationLimit=inf  LowerSaturationLimit=-inf  LinearizeAsGain=off  AntiWindupMode=none  Kb=1  TrackingMode=off  Kt=1  PParamMin=[]  PParamMax=[]  IParamMin=[]  IParamMax=[]  DParamMin=[]  DParamMax=[]  NParamMin=[]  NParamMax=[]  bParamMin=[]  bParamMax=[]  cParamMin=[]  cParamMax=[]  KbParamMin=[]  KbParamMax=[]  KtParamMin=[]  KtParamMax=[]  POutMin=[]  POutMax=[]  IOutMin=[]  IOutMax=[]  DOutMin=[]  DOutMax=[]  NOutMin=[]  NOutMax=[]  bOutMin=[]  bOutMax=[]  cOutMin=[]  cOutMax=[]  KbOutMin=[]  KbOutMax=[]  KtOutMin=[]  KtOutMax=[]  IntegratorOutMin=[]  IntegratorOutMax=[]  FilterOutMin=[]  FilterOutMax=[]  SumOutMin=[]  SumOutMax=[]  Sum1OutMin=[]  Sum1OutMax=[]  Sum2OutMin=[]  Sum2OutMax=[]  Sum3OutMin=[]  Sum3OutMax=[]  SumI1OutMin=[]  SumI1OutMax=[]  SumI2OutMin=[]  SumI2OutMax=[]  SumI3OutMin=[]  SumI3OutMax=[]  SumDOutMin=[]  SumDOutMax=[]  SaturationOutMin=[]  SaturationOutMax=[]  IntegratorContinuousStateAttributes=''  IntegratorStateMustResolveToSignalObject=off  IntegratorRTWStateStorageClass=Auto  FilterContinuousStateAttributes=''  FilterStateMustResolveToSignalObject=off  FilterRTWStateStorageClass=Auto  DifferentiatorICPrevScaledInput=0  DifferentiatorOutMin=[]  DifferentiatorOutMax=[]  FilterDiffOutCoefMin=[]  FilterDiffOutCoefMax=[]  SumDenOutMin=[]  SumDenOutMax=[]  SumNumOutMin=[]  SumNumOutMax=[]  ReciprocalOutMin=[]  ReciprocalOutMax=[]  DivideOutMin=[]  DivideOutMax=[]  TunerSelectOption=Transfer Function Based (PID Tuner App)
  cyemi_{448..456} (9 alike) : DataTypeConversion  OutDataTypeStr=double
  cfblk2 : Outport
  cfblk14 : Outport  Port=2
  cfblk15 : Outport  Port=3
  wires:
  cfblk3/1 -> cfblk2/1
  cfblk11/1 -> cfblk14/1
  cfblk9/1 -> cfblk15/1
  cyemi_448/1 -> cfblk10/1
  cfblk12/1 -> cyemi_448/1
  cyemi_449/1 -> cfblk3/1
  cfblk5/1 -> cyemi_449/1
  cyemi_450/1 -> cfblk4/1
  cfblk10/1 -> cyemi_450/1
  cyemi_451/1 -> cfblk5/1
  cfblk6/1 -> cyemi_451/1
  cyemi_452/1 -> cfblk6/1
  cfblk8/1 -> cyemi_452/1
  cyemi_453/1 -> cfblk7/1
  cfblk1/1 -> cyemi_453/1
  cyemi_454/1 -> cfblk8/1
  cfblk13/1 -> cyemi_454/1
  cyemi_455/1 -> cfblk9/1
  cfblk7/1 -> cyemi_455/1
  cyemi_456/1 -> cfblk9/2
  cfblk4/1 -> cyemi_456/1
